simulink model "TRMS_sim"  (R2021a)
settings: Solver=VariableStepAuto  StartTime=0.0  StopTime=100  MaxStep=1e-2  RelTol=1e-3
undefined symbols (not defined in the file or in its folder): qLPV_TRMS_SS_sim, TRMS
settings Model: Creator=ariel  LastModifiedBy=ariel

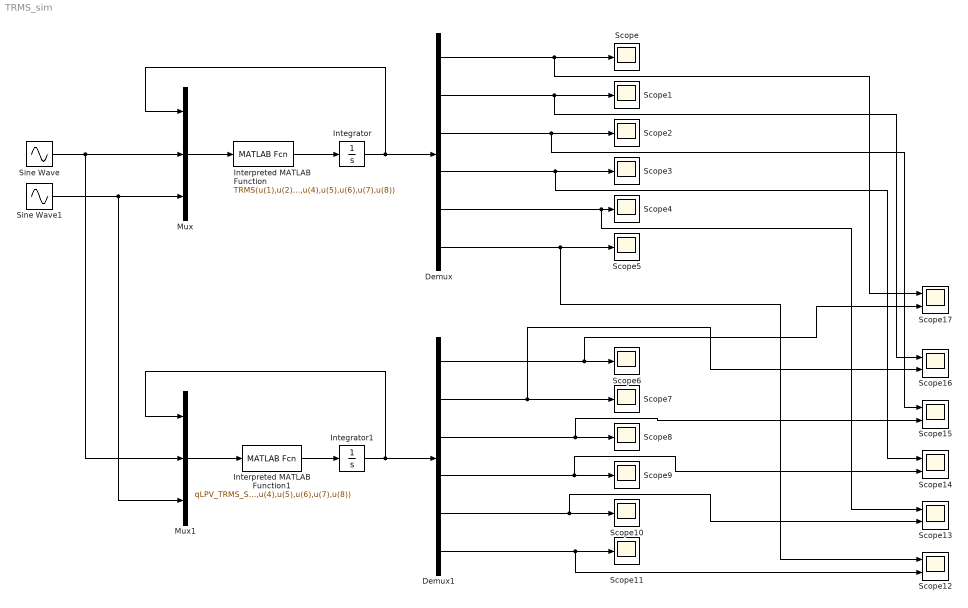
== system TRMS_sim ==
  Demux : Demux  Outputs=6
  Demux1 : Demux  Outputs=6
  Integrator : Integrator
  Integrator1 : Integrator  InitialCondition=[0 0 0 0 0 0]'
  Interpreted MATLAB Function : MATLABFcn  MATLABFcn=TRMS(u(1),u(2),u(3),u(4),u(5),u(6),u(7),u(8))  OutputDimensions=6
  Interpreted MATLAB Function1 : MATLABFcn  MATLABFcn=qLPV_TRMS_SS_sim(u(1),u(2),u(3),u(4),u(5),u(6),u(7),u(8))  OutputDimensions=6
  Mux : Mux  Inputs=3
  Mux1 : Mux  Inputs=3
  Scope{,1..11} (12 alike) : Scope
  Scope{12..17} (6 alike) : Scope  NumInputPorts=2
  Sine Wave : Sin  Frequency=2*pi*(1/10)  Phase=0.5  SampleTime=0
  Sine Wave1 : Sin  Frequency=2*pi*(1/15)  Phase=0.3  SampleTime=0
  wires:
  Interpreted MATLAB Function/1 -> Integrator/1
  Mux/1 -> Interpreted MATLAB Function/1
  Integrator/1 -> Demux/1, Mux/1
  Demux/1 -> Scope17/1, Scope/1
  Demux/6 -> Scope12/1, Scope5/1
  Demux/5 -> Scope13/1, Scope4/1
  Demux/4 -> Scope14/1, Scope3/1
  Demux/3 -> Scope15/1, Scope2/1
  Demux/2 -> Scope16/1, Scope1/1
  Demux1/2 -> Scope16/2, Scope7/1
  Demux1/3 -> Scope15/2, Scope8/1
  Demux1/4 -> Scope14/2, Scope9/1
  Demux1/1 -> Scope17/2, Scope6/1
  Sine Wave1/1 -> Mux1/3, Mux/3
  Demux1/5 -> Scope13/2, Scope10/1
  Integrator1/1 -> Demux1/1, Mux1/1
  Sine Wave/1 -> Mux1/2, Mux/2
  Interpreted MATLAB Function1/1 -> Integrator1/1
  Mux1/1 -> Interpreted MATLAB Function1/1
  Demux1/6 -> Scope12/2, Scope11/1
